simulink model "SIM"  (R2013b)
settings: Solver=ode45  StartTime=0.0  StopTime=10.0  RelTol=1e-3
libraries: nesl_utility x11, pe_lib x10, fl_lib x7, simulink x3, powerlib_meascontrol x3
settings Model: Creator=Eduardo  LastModifiedBy=Eduardo

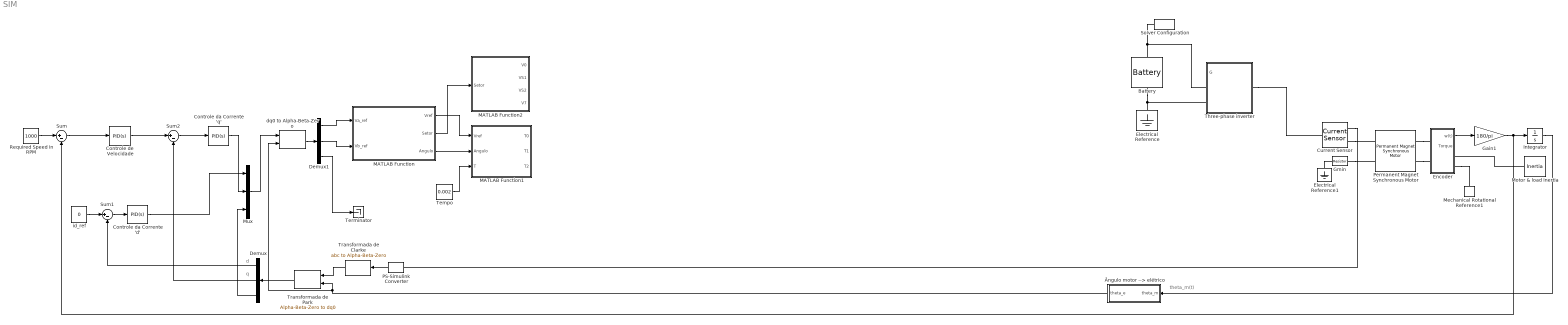
== system SIM ==
  note: d
  note: q
  note: theta_m(t)
  Battery : pe_lib/Sources/Battery  Vnom=12 V  AH=14000 hr*A  AH0=7000 hr*A  V1=470 V  AH1=5000 hr*A  R1=0.001 Ohm  R2=inf Ohm  alpha=1  beta=1  G2=0 S  i_Log=off  charge_Log=off  LocalVarNames=|i|charge  LocalVarDescs=|i|Charge state  LocalVarLogging=[0 0]
  Controle da Corrente 'q' : simulink/Continuous/PID Controller  Controller=PID  TimeDomain=Continuous-time  SampleTime=1  IntegratorMethod=Forward Euler  FilterMethod=Forward Euler  Form=Parallel  P=1  I=1  D=0  N=100  InitialConditionSource=internal  InitialConditionForIntegrator=0  InitialConditionForFilter=0  ExternalReset=none  LimitOutput=off  UpperSaturationLimit=inf  LowerSaturationLimit=-inf  LinearizeAsGain=on  AntiWindupMode=none  Kb=1  TrackingMode=off  Kt=1  PParamMin=[]  PParamMax=[]  IParamMin=[]  IParamMax=[]  DParamMin=[]  DParamMax=[]  NParamMin=[]  NParamMax=[]  KbParamMin=[]  KbParamMax=[]  KtParamMin=[]  KtParamMax=[]  POutMin=[]  POutMax=[]  IOutMin=[]  IOutMax=[]  DOutMin=[]  DOutMax=[]  NOutMin=[]  NOutMax=[]  KbOutMin=[]  KbOutMax=[]  KtOutMin=[]  KtOutMax=[]  IntegratorOutMin=[]  IntegratorOutMax=[]  FilterOutMin=[]  FilterOutMax=[]  SumOutMin=[]  SumOutMax=[]  SumI1OutMin=[]  SumI1OutMax=[]  SumI2OutMin=[]  SumI2OutMax=[]  SumI3OutMin=[]  SumI3OutMax=[]  SumDOutMin=[]  SumDOutMax=[]  SaturationOutMin=[]  SaturationOutMax=[]  IntegratorContinuousStateAttributes=''  IntegratorStateMustResolveToSignalObject=off  IntegratorRTWStateStorageClass=Auto  FilterContinuousStateAttributes=''  FilterStateMustResolveToSignalObject=off  FilterRTWStateStorageClass=Auto
  Controle da Corrente 'd' : simulink/Continuous/PID Controller  Controller=PID  TimeDomain=Continuous-time  SampleTime=1  IntegratorMethod=Forward Euler  FilterMethod=Forward Euler  Form=Parallel  P=1  I=1  D=0  N=100  InitialConditionSource=internal  InitialConditionForIntegrator=0  InitialConditionForFilter=0  ExternalReset=none  LimitOutput=off  UpperSaturationLimit=inf  LowerSaturationLimit=-inf  LinearizeAsGain=on  AntiWindupMode=none  Kb=1  TrackingMode=off  Kt=1  PParamMin=[]  PParamMax=[]  IParamMin=[]  IParamMax=[]  DParamMin=[]  DParamMax=[]  NParamMin=[]  NParamMax=[]  KbParamMin=[]  KbParamMax=[]  KtParamMin=[]  KtParamMax=[]  POutMin=[]  POutMax=[]  IOutMin=[]  IOutMax=[]  DOutMin=[]  DOutMax=[]  NOutMin=[]  NOutMax=[]  KbOutMin=[]  KbOutMax=[]  KtOutMin=[]  KtOutMax=[]  IntegratorOutMin=[]  IntegratorOutMax=[]  FilterOutMin=[]  FilterOutMax=[]  SumOutMin=[]  SumOutMax=[]  SumI1OutMin=[]  SumI1OutMax=[]  SumI2OutMin=[]  SumI2OutMax=[]  SumI3OutMin=[]  SumI3OutMax=[]  SumDOutMin=[]  SumDOutMax=[]  SaturationOutMin=[]  SaturationOutMax=[]  IntegratorContinuousStateAttributes=''  IntegratorStateMustResolveToSignalObject=off  IntegratorRTWStateStorageClass=Auto  FilterContinuousStateAttributes=''  FilterStateMustResolveToSignalObject=off  FilterRTWStateStorageClass=Auto
  Controle de Velocidade : simulink/Continuous/PID Controller  Controller=PID  TimeDomain=Continuous-time  SampleTime=1  IntegratorMethod=Forward Euler  FilterMethod=Forward Euler  Form=Parallel  P=1  I=1  D=0  N=100  InitialConditionSource=internal  InitialConditionForIntegrator=0  InitialConditionForFilter=0  ExternalReset=none  LimitOutput=off  UpperSaturationLimit=inf  LowerSaturationLimit=-inf  LinearizeAsGain=on  AntiWindupMode=none  Kb=1  TrackingMode=off  Kt=1  PParamMin=[]  PParamMax=[]  IParamMin=[]  IParamMax=[]  DParamMin=[]  DParamMax=[]  NParamMin=[]  NParamMax=[]  KbParamMin=[]  KbParamMax=[]  KtParamMin=[]  KtParamMax=[]  POutMin=[]  POutMax=[]  IOutMin=[]  IOutMax=[]  DOutMin=[]  DOutMax=[]  NOutMin=[]  NOutMax=[]  KbOutMin=[]  KbOutMax=[]  KtOutMin=[]  KtOutMax=[]  IntegratorOutMin=[]  IntegratorOutMax=[]  FilterOutMin=[]  FilterOutMax=[]  SumOutMin=[]  SumOutMax=[]  SumI1OutMin=[]  SumI1OutMax=[]  SumI2OutMin=[]  SumI2OutMax=[]  SumI3OutMin=[]  SumI3OutMax=[]  SumDOutMin=[]  SumDOutMax=[]  SaturationOutMin=[]  SaturationOutMax=[]  IntegratorContinuousStateAttributes=''  IntegratorStateMustResolveToSignalObject=off  IntegratorRTWStateStorageClass=Auto  FilterContinuousStateAttributes=''  FilterStateMustResolveToSignalObject=off  FilterRTWStateStorageClass=Auto
  Current Sensor : pe_lib/Sensors/Current Sensor  I_Log=off  LocalVarNames=|i_a|i_b|i_c  LocalVarDescs=|i_a|i_b|i_c  LocalVarLogging=[0 0 0]  i_a_Log=off  i_b_Log=off  i_c_Log=off
  Demux : Demux  Outputs=3
  Demux1 : Demux  Outputs=3
  Electrical Reference : fl_lib/Electrical/Electrical Elements/Electrical Reference  i_Log=off  LocalVarNames=|i  LocalVarDescs=|i  LocalVarLogging=0
  Electrical Reference1 : fl_lib/Electrical/Electrical Elements/Electrical Reference  i_Log=off  LocalVarNames=|i  LocalVarDescs=|i  LocalVarLogging=0
  Encoder : Subsystem
  Gain1 : Gain  Gain=180/pi
  Gmin : fl_lib/Electrical/Electrical Elements/Resistor  R=1e9 Ohm  i_Log=off  v_Log=off  LocalVarNames=|i|v  LocalVarDescs=|i|v  LocalVarLogging=[0 0]
  Integrator : Integrator
  MATLAB Function : MATLAB Function  TreatAsAtomicUnit=on
  MATLAB Function1 : MATLAB Function  TreatAsAtomicUnit=on
  MATLAB Function2 : MATLAB Function  TreatAsAtomicUnit=on
  Mechanical Rotational Reference1 : fl_lib/Mechanical/Rotational Elements/Mechanical Rotational Reference  t_Log=off  LocalVarNames=|t  LocalVarDescs=|t  LocalVarLogging=0
  Motor & load inertia : fl_lib/Mechanical/Rotational Elements/Inertia  inertia=10 kg*m^2  initial_velocity=0 rpm  t_Log=off  LocalVarNames=|t  LocalVarDescs=|t  LocalVarLogging=0
  Mux : Mux  Inputs=3
  PS-Simulink Converter : nesl_utility/PS-Simulink Converter  PhysicalDomain=network_engine_domain  SubClassName=ps_output  LeftPortType=input  RightPortType=output  PseudoPeriodic=off  Frequencies=[]  Unit=A  AffineConversion=off
  Permanent Magnet Synchronous Motor : pe_lib/Machines/Permanent Magnet Rotor/Permanent Magnet Synchronous Motor  nPolePairs=6  pm_flux_linkage=0.03 Wb  stator_param=1  Ld=0.00025 H  Lq=0.00019 H  L0=0.00016 H  Ls=0.0002 H  Lm=0.00002 H  Ms=0.00002 H  Rs=0.013 Ohm  initial_currents=[0, 0, 0] A  axes_param=2  angular_position0=0 deg  LocalVarNames=|i_d|i_q|i_0|v_a|v_b|v_c|i_a|i_b|i_c|i_n|torque|angular_velocity|angular_position  LocalVarDescs=|i_d|i_q|i_0|v_a|v_b|v_c|i_a|i_b|i_c|i_n|torque|angular_velocity|angular_position  LocalVarLogging=[0 0 0 0 0 0 0 0 0 0 0 0 0]  rotor_offset=- pi / 2 rad  shift_3ph=[nan, nan, nan] rad  sqrt2OverSqrt3=nan  oneOverSqrt2=nan  twoPiOver3=nan  Lmin=1e-9 H  i_d_Log=off  i_q_Log=off  i_0_Log=off  v_a_Log=off  v_b_Log=off  v_c_Log=off  i_a_Log=off  i_b_Log=off  i_c_Log=off  i_n_Log=off  torque_Log=off  angular_velocity_Log=off  angular_position_Log=off
  "Required Speed in RPM " : Constant  Value=1000
  Solver Configuration : nesl_utility/Solver Configuration  PhysicalDomain=network_engine_domain  SubClassName=solver  LeftPortType=input  RightPortType=generic  Accelerate=off  Tones=[]  Harmonics=[]  SimulateNoise=off  Profile=off  UseLocalSampling=off  EnableSwitchedLinearOptims=on  FrequencyDomain=off  UseCCode=off  RelTol=0.001  AbsTol=1e-06  MinStep=1e-09  ToWorkspace=off  DoDC=off  ResidualTolerance=1e-9  UseLocalSolver=on  LocalSolverChoice=NE_BACKWARD_EULER_ADVANCER  LocalSolverSampleTime=1e-5  DoFixedCost=on  MaxNonlinIter=3  MaxModeIter=2  LinearAlgebra=Sparse  DelaysMemoryBudget=1024
  Sum : Sum  Inputs=|+-
  Sum1 : Sum  Inputs=|+-
  Sum2 : Sum  Inputs=|+-
  "Tempo " : Constant  Value=0.002
  Terminator : Terminator
  Three-phase inverter : Subsystem
  Transformada de Park : powerlib_meascontrol/Transformations/Alpha-Beta-Zero to dq0  Alignment=90 degrees behind phase A axis
  Transformada de Clarke : powerlib_meascontrol/Transformations/abc to Alpha-Beta-Zero
  dq0 to Alpha-Beta-Zero : powerlib_meascontrol/Transformations/dq0 to Alpha-Beta-Zero  Alignment=90 degrees behind phase A axis
  "id_ref " : Constant  Value=0
  Ângulo motor --> elétrico : Subsystem
  wires:
  "Required Speed in RPM "/1 -> Sum/1
  PS-Simulink Converter/1 -> Transformada de Clarke/1
  Encoder/1(w(t)) -> Gain1/1
  Integrator/1 -> Ângulo motor --> elétrico/1(theta_m)
  Transformada de Clarke/1 -> Transformada de Park/1
  Ângulo motor --> elétrico/1(theta_e) -> dq0 to Alpha-Beta-Zero/2, Transformada de Park/2
  Transformada de Park/1 -> Demux/1
  Demux/1 -> Sum1/2
  Demux/2 -> Sum2/2
  "id_ref "/1 -> Sum1/1
  Sum1/1 -> Controle da Corrente 'd'/1
  Gain1/1 -> Integrator/1, Sum/2
  Sum/1 -> Controle de Velocidade/1
  Controle de Velocidade/1 -> Sum2/1
  Sum2/1 -> Controle da Corrente 'q'/1
  Controle da Corrente 'd'/1 -> Mux/1
  Controle da Corrente 'q'/1 -> Mux/2
  Demux/3 -> Mux/3
  Mux/1 -> dq0 to Alpha-Beta-Zero/1
  dq0 to Alpha-Beta-Zero/1 -> Demux1/1
  Demux1/1 -> MATLAB Function/1(Va_ref)
  Demux1/2 -> MATLAB Function/2(Vb_ref)
  Demux1/3 -> Terminator/1
  MATLAB Function/1(Vref) -> MATLAB Function1/1(Vref)
  MATLAB Function/3(Angulo) -> MATLAB Function1/2(Angulo)
  "Tempo "/1 -> MATLAB Function1/3(T)
  MATLAB Function/2(Setor) -> MATLAB Function2/1(Setor)
  connections:
  Current Sensor/RConn2 -- Permanent Magnet Synchronous Motor/LConn1
  Electrical Reference1/LConn1 -- Gmin/LConn1
  Gmin/RConn1 -- Permanent Magnet Synchronous Motor/LConn2
  Current Sensor/RConn1 -- PS-Simulink Converter/LConn1
  Permanent Magnet Synchronous Motor/RConn2 -- Encoder/LConn2
  Permanent Magnet Synchronous Motor/RConn1 -- Encoder/LConn1
  Encoder/RConn2 -- Mechanical Rotational Reference1/LConn1
  Motor & load inertia/LConn1 -- Encoder/RConn1
  Solver Configuration/RConn1 -- Battery/LConn1 -- Three-phase inverter/LConn1
  Electrical Reference/LConn1 -- Battery/RConn1 -- Three-phase inverter/LConn2
  Three-phase inverter/RConn1 -- Current Sensor/LConn1

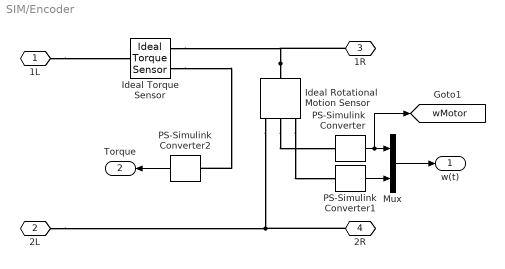
== system SIM/Encoder ==
  Ideal Rotational Motion Sensor : fl_lib/Mechanical/Mechanical Sensors/Ideal Rotational Motion Sensor  offset=0 deg  w_Log=off  t_Log=off  phi_Log=off  LocalVarNames=|w|t|phi  LocalVarDescs=|w|t|phi  LocalVarLogging=[0 0 0]
  Ideal Torque Sensor : fl_lib/Mechanical/Mechanical Sensors/Ideal Torque Sensor  w_Log=off  t_Log=off  LocalVarNames=|w|t  LocalVarDescs=|w|t  LocalVarLogging=[0 0]
  Mux : Mux  Inputs=2
  PS-Simulink Converter : nesl_utility/PS-Simulink Converter  PhysicalDomain=network_engine_domain  SubClassName=ps_output  LeftPortType=input  RightPortType=output  PseudoPeriodic=off  Frequencies=[]  Unit=rad/s  AffineConversion=off
  PS-Simulink Converter1 : nesl_utility/PS-Simulink Converter  PhysicalDomain=network_engine_domain  SubClassName=ps_output  LeftPortType=input  RightPortType=output  PseudoPeriodic=off  Frequencies=[]  Unit=rad  AffineConversion=off
  PS-Simulink Converter2 : nesl_utility/PS-Simulink Converter  PhysicalDomain=network_engine_domain  SubClassName=ps_output  LeftPortType=input  RightPortType=output  PseudoPeriodic=off  Frequencies=[]  Unit=N*m  AffineConversion=off
  1L : PMIOPort  Port=1  Side=Left
  2L : PMIOPort  Port=2  Side=Left
  1R : PMIOPort  Port=3  Side=Right
  2R : PMIOPort  Port=4  Side=Right
  w(t) : Outport
  Torque : Outport  Port=2
  tag scope: wMotor=global
  wires:
  PS-Simulink Converter2/1 -> Torque/1
  Mux/1 -> w(t)/1
  PS-Simulink Converter1/1 -> Mux/2
  PS-Simulink Converter/1 -> [wMotor], Mux/1
  connections:
  Ideal Torque Sensor/RConn2 -- PS-Simulink Converter2/LConn1
  1L/RConn1 -- Ideal Torque Sensor/LConn1
  2R/RConn1 -- 2L/RConn1 -- Ideal Rotational Motion Sensor/RConn1
  Ideal Rotational Motion Sensor/LConn1 -- 1R/RConn1 -- Ideal Torque Sensor/RConn1
  Ideal Rotational Motion Sensor/RConn2 -- PS-Simulink Converter/LConn1
  Ideal Rotational Motion Sensor/RConn3 -- PS-Simulink Converter1/LConn1

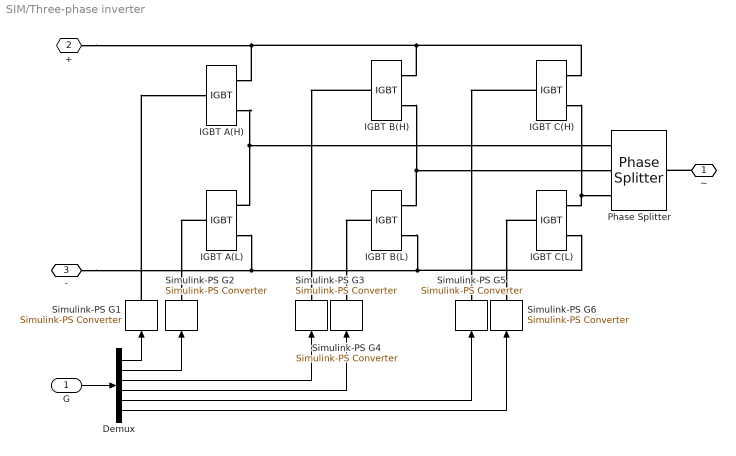
== system SIM/Three-phase inverter ==
  G : Inport
  Demux : Demux  Outputs=6
  IGBT A(H) : pe_lib/Semiconductors/Fundamental Components/IGBT  Vf=0.8 V  Ron=0.001 Ohm  Goff=1e-5 S  Vth=0.5 V  diode_param=2  diode_Vf=0.8 V  diode_Ron=0.001 Ohm  diode_Goff=1e-5 S  diode_C=5e-8 F  diode_iRM=-235 A  diode_iF=300 A  diode_idot=-50 A/us  diode_trr_param=1  diode_trr_factor=3  diode_trr=15 us  diode_Qrr=1.5e+3 s*uA  LocalVarLogging=[]
  IGBT A(L) : pe_lib/Semiconductors/Fundamental Components/IGBT  Vf=0.8 V  Ron=0.001 Ohm  Goff=1e-5 S  Vth=0.5 V  diode_param=2  diode_Vf=0.8 V  diode_Ron=0.001 Ohm  diode_Goff=1e-5 S  diode_C=5e-8 F  diode_iRM=-235 A  diode_iF=300 A  diode_idot=-50 A/us  diode_trr_param=1  diode_trr_factor=3  diode_trr=15 us  diode_Qrr=1.5e+3 s*uA  LocalVarLogging=[]
  IGBT B(H) : pe_lib/Semiconductors/Fundamental Components/IGBT  Vf=0.8 V  Ron=0.001 Ohm  Goff=1e-5 S  Vth=0.5 V  diode_param=2  diode_Vf=0.8 V  diode_Ron=0.001 Ohm  diode_Goff=1e-5 S  diode_C=5e-8 F  diode_iRM=-235 A  diode_iF=300 A  diode_idot=-50 A/us  diode_trr_param=1  diode_trr_factor=3  diode_trr=15 us  diode_Qrr=1.5e+3 s*uA  LocalVarLogging=[]
  IGBT B(L) : pe_lib/Semiconductors/Fundamental Components/IGBT  Vf=0.8 V  Ron=0.001 Ohm  Goff=1e-5 S  Vth=0.5 V  diode_param=2  diode_Vf=0.8 V  diode_Ron=0.001 Ohm  diode_Goff=1e-5 S  diode_C=5e-8 F  diode_iRM=-235 A  diode_iF=300 A  diode_idot=-50 A/us  diode_trr_param=1  diode_trr_factor=3  diode_trr=15 us  diode_Qrr=1.5e+3 s*uA  LocalVarLogging=[]
  IGBT C(H) : pe_lib/Semiconductors/Fundamental Components/IGBT  Vf=0.8 V  Ron=0.001 Ohm  Goff=1e-5 S  Vth=0.5 V  diode_param=2  diode_Vf=0.8 V  diode_Ron=0.001 Ohm  diode_Goff=1e-5 S  diode_C=5e-8 F  diode_iRM=-235 A  diode_iF=300 A  diode_idot=-50 A/us  diode_trr_param=1  diode_trr_factor=3  diode_trr=15 us  diode_Qrr=1.5e+3 s*uA  LocalVarLogging=[]
  IGBT C(L) : pe_lib/Semiconductors/Fundamental Components/IGBT  Vf=0.8 V  Ron=0.001 Ohm  Goff=1e-5 S  Vth=0.5 V  diode_param=2  diode_Vf=0.8 V  diode_Ron=0.001 Ohm  diode_Goff=1e-5 S  diode_C=5e-8 F  diode_iRM=-235 A  diode_iF=300 A  diode_idot=-50 A/us  diode_trr_param=1  diode_trr_factor=3  diode_trr=15 us  diode_Qrr=1.5e+3 s*uA  LocalVarLogging=[]
  Phase Splitter : pe_lib/Connections/Phase Splitter  I_Log=off  i_a_Log=off  i_b_Log=off  i_c_Log=off  LocalVarNames=|I|i_a|i_b|i_c  LocalVarDescs=|I|i_a|i_b|i_c  LocalVarLogging=[0 0 0 0]
  Simulink-PS G{1..6} (6 alike) : nesl_utility/Simulink-PS Converter  PhysicalDomain=network_engine_domain  SubClassName=ps_input  LeftPortType=input  RightPortType=output  PseudoPeriodic=off  Frequencies=[]  NoiseDistribution=none  NoiseParameters=[]  Unit=1  AffineConversion=off  InputFiltering=off  SimscapeFilterOrder=1  InputFilterTimeConstant=1e-6  UdotUserProvided=0
  ~ : PMIOPort  Tag=PMCPort  Port=1  Side=Right
  + : PMIOPort  Tag=PMCPort  Port=2  Side=Left
  - : PMIOPort  Tag=PMCPort  Port=3  Side=Left
  wires:
  Demux/6 -> Simulink-PS G6/1
  Demux/5 -> Simulink-PS G5/1
  Demux/4 -> Simulink-PS G4/1
  Demux/3 -> Simulink-PS G3/1
  Demux/2 -> Simulink-PS G2/1
  G/1 -> Demux/1
  Demux/1 -> Simulink-PS G1/1
  connections:
  IGBT C(L)/LConn1 -- Simulink-PS G6/RConn1
  IGBT C(H)/LConn1 -- Simulink-PS G5/RConn1
  IGBT B(L)/LConn1 -- Simulink-PS G4/RConn1
  IGBT B(H)/LConn1 -- Simulink-PS G3/RConn1
  IGBT A(L)/LConn1 -- Simulink-PS G2/RConn1
  -/RConn1 -- IGBT A(L)/RConn2 -- IGBT C(L)/RConn2 -- IGBT B(L)/RConn2
  IGBT A(H)/RConn2 -- IGBT A(L)/RConn1 -- Phase Splitter/RConn1
  IGBT B(L)/RConn1 -- IGBT B(H)/RConn2 -- Phase Splitter/RConn2
  IGBT C(L)/RConn1 -- IGBT C(H)/RConn2 -- Phase Splitter/RConn3
  +/RConn1 -- IGBT A(H)/RConn1 -- IGBT C(H)/RConn1 -- IGBT B(H)/RConn1
  ~/RConn1 -- Phase Splitter/LConn1
  Simulink-PS G1/RConn1 -- IGBT A(H)/LConn1

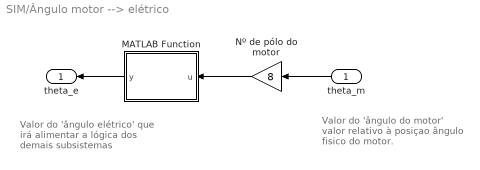
== system SIM/Ângulo motor --> elétrico ==
  note: Valor do 'ângulo do motor'
      | valor relativo à posiçao
      | ângulo fisico do motor.
  note: Valor do 'ângulo elétrico'
      | que irá alimentar a lógica
      | dos demais subsistemas
  theta_m : Inport
  MATLAB Function : MATLAB Function  TreatAsAtomicUnit=on
  Nº de pólo do motor : Gain  Gain=8
  theta_e : Outport
  wires:
  theta_m/1 -> Nº de pólo do motor/1
  MATLAB Function/1(y) -> theta_e/1
  Nº de pólo do motor/1 -> MATLAB Function/1(u)

== matlab function SIM/MATLAB Function ==
  data: Va_ref input; Vref output; Vb_ref input; Setor output; Angulo output
function [Vref, Setor, Angulo] = AfterInverseClarkeTransform(Va_ref, Vb_ref)

%%% 1º Módulo
Vref = sqrt(Valfa_ref^2 + Vbeta_ref^2);

%%% 2º Ângulo para definição do setor
Ang = atan2(Vb_ref, Va_ref);
Ang = Ang*180/pi;
Ang = mod(Ang,360);

if ((Ang >= 0) && (Ang <60))
    Setor = 1;
elseif((Ang >= 60) && (Ang <120))
    Setor = 2;
elseif((Ang >= 120) && (Ang <180))
    Setor = 3;
elseif((Ang >= 180) && (Ang <240))
    Setor = 4;
elseif((Ang >= 240) && (Ang <=300))
    Setor = 5;
elseif((Ang >= 300) && (Ang <360))
    Setor = 6;
elseif (Ang == 360)
    Setor = 1;
end

%%% 3º Ângulo no setor (em radiano)
Angulo = mod(Ang, 60)*pi/180;



end

== matlab function SIM/Ângulo motor --> elétrico/MATLAB Function ==
  data: u input; y output
function y = satura360(u)

% A resposta do ângulo se dará em 'radianos'.
y = mod(u,360)*pi/180;

== matlab function SIM/MATLAB Function1 ==
  data: Vref input; T0 output; Angulo input; T input; T1 output; T2 output
function [T0, T1, T2] = Times(Vref, Angulo, T)

T1 = T*Vref*2*sin((pi/3) - Angulo)/sqrt(3);   % Tempo para o V1.
T2 = T*Vref*2*sin(Angulo)/sqrt(3);            % Tempo para o V2.
T0 = T - T1 - T2;                             % Tempo para o Vetor Nulo.

end

== matlab function SIM/MATLAB Function2 ==
  data: Setor input; V0 output; VS1 output; VS2 output; V7 output
function [V0, VS1, VS2, V7] = Uxxx(Setor)

V0 = [0 0 0];
V1 = [1 0 0];
V2 = [1 1 0];
V3 = [0 1 0];
V4 = [0 1 1];
V5 = [0 0 1];
V6 = [1 0 1];
V7 = [1 1 1];

if (Setor == 1)
    VS1 = V1;
    VS2 = V2;
elseif (Setor == 2)
    VS1 = V2;
    VS2 = V3;
elseif (Setor == 3)
    VS1 = V3;
    VS2 = V4;
elseif (Setor == 4)
    VS1 = V4;
    VS2 = V5; 
elseif (Setor ==5)
    VS1 = V5;
    VS2 = V6;   
elseif (Setor == 6)
    VS1 = V6;
    VS2 = V1;
end

end
